simulink model "Demo1"  (R2018b)
settings: Solver=FixedStepDiscrete  StartTime=0.0  StopTime=10  FixedStep=0.0005  RelTol=1e-3  EnableMultiTasking=on
undefined symbols (not defined in the file or in its folder): ADS1, ADS2, br_opening, BRAKE, I_AN06_5V, I_AN08_5V, I_AN09_5V, I_AN10_5V, I_HALL1, I_HALL2, I_SW11_H, I_SW16_H, MnPedal_H, MnPedal_L, MxPedal_H, MxPedal_L, O_PWM1_LS0A7, O_PWM2_LS0A7, O_SW02_LS0A4, O_SW13_HS1A, O_SW14_HS1A, PUMP, th_opening
libraries: ec5744lib x93, canmsglib x14, simulink x5
(part 2 of 2)

== system Demo1/Function-Call Subsystem1/Subsystem ==
  note: 油压范围在500到4500之间
  note: 输出12V高电平给蜂鸣器和待驶指示
      | 灯，启动鸣笛，指示灯亮
  Brake : Inport  OutDataTypeStr=uint16
  Key : Inport  Port=2
  MCU1_rdy : Inport  Port=3
  MCU2_rdy : Inport  Port=4
  1-D Lookup Table2 : Lookup_n-D  NumberOfTableDimensions=1  BreakpointsForDimension1=BRAKE  Table=br_opening  ExtrapMethod=Clip  InternalRulePriority=Speed  OutMin=0  OutMax=100  OutDataTypeStr=uint8  RndMeth=Simplest  InputSameDT=on
  MeaModule3 : ec5744lib/RapidECU_U3/07Calibration/MeaModule  signal=RS
      settings: SourceProductName=ECUCoder for MPC5744
  Terminator : Terminator
  WaitStart&Brake_LED : Stateflow chart  TreatAsAtomicUnit=on
  Break_LED : Outport
  WS_Sig : Outport  Port=2
  WAIT_START : Outport  Port=3
  wires:
  WaitStart&Brake_LED/1(Wait_Start) -> WAIT_START/1  "Wait_Start"
  Brake/1 -> 1-D Lookup Table2/1
  1-D Lookup Table2/1 -> WaitStart&Brake_LED/1(Brake)
  WaitStart&Brake_LED/2(Break_LED) -> Break_LED/1  "Break_LED"
  Key/1 -> WaitStart&Brake_LED/2(Key)
  WaitStart&Brake_LED/3(WS_Sig) -> WS_Sig/1
  WaitStart&Brake_LED/4(RS) -> MeaModule3/1
  MeaModule3/1 -> Terminator/1
  MCU1_rdy/1 -> WaitStart&Brake_LED/3(MCU1_rdy)
  MCU2_rdy/1 -> WaitStart&Brake_LED/4(MCU2_rdy)

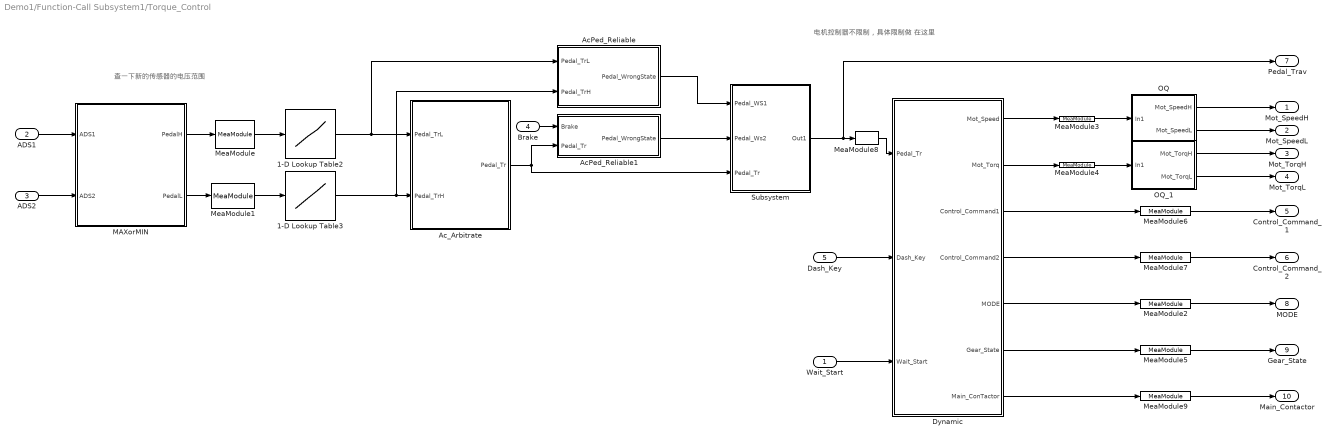
== system Demo1/Function-Call Subsystem1/Torque_Control ==
  note: 查一下新的传感器的电压范围
  note: 电机控制器不限制，具体限制做
      | 在这里
  Wait_Start : Inport
  ADS1 : Inport  Port=2
  ADS2 : Inport  Port=3  OutDataTypeStr=uint16
  "Brake " : Inport  Port=4
  "Dash_Key " : Inport  Port=5  OutMin=0  OutMax=2
  1-D Lookup Table2 : Lookup_n-D  NumberOfTableDimensions=1  BreakpointsForDimension1=ADS1  Table=th_opening  ExtrapMethod=Clip  InternalRulePriority=Speed  OutMin=0  OutMax=95  OutDataTypeStr=uint8  RndMeth=Simplest  InputSameDT=on
  1-D Lookup Table3 : Lookup_n-D  NumberOfTableDimensions=1  BreakpointsForDimension1=ADS2  Table=th_opening  ExtrapMethod=Clip  InternalRulePriority=Speed  OutMin=0  OutMax=95  OutDataTypeStr=uint8  RndMeth=Simplest  InputSameDT=on
  AcPed_Reliable : Stateflow chart  TreatAsAtomicUnit=on
  AcPed_Reliable1 : Stateflow chart  TreatAsAtomicUnit=on
  Ac_Arbitrate : Stateflow chart  TreatAsAtomicUnit=on
  "Dynamic " : Stateflow chart  TreatAsAtomicUnit=on
  MAXorMIN : Subsystem
  MeaModule : ec5744lib/RapidECU_U3/07Calibration/MeaModule  signal=ADSH
      settings: SourceProductName=ECUCoder for MPC5744
  MeaModule1 : ec5744lib/RapidECU_U3/07Calibration/MeaModule  signal=ADSL
      settings: SourceProductName=ECUCoder for MPC5744
  MeaModule2 : ec5744lib/RapidECU_U3/07Calibration/MeaModule  signal=MODE
      settings: SourceProductName=ECUCoder for MPC5744
  MeaModule3 : ec5744lib/RapidECU_U3/07Calibration/MeaModule  signal=MotSpeed
      settings: SourceProductName=ECUCoder for MPC5744
  MeaModule4 : ec5744lib/RapidECU_U3/07Calibration/MeaModule  signal=Mot_torq
      settings: SourceProductName=ECUCoder for MPC5744
  MeaModule5 : ec5744lib/RapidECU_U3/07Calibration/MeaModule  signal=Gear_State
      settings: SourceProductName=ECUCoder for MPC5744
  MeaModule6 : ec5744lib/RapidECU_U3/07Calibration/MeaModule  signal=Control1
      settings: SourceProductName=ECUCoder for MPC5744
  MeaModule7 : ec5744lib/RapidECU_U3/07Calibration/MeaModule  signal=Control2
      settings: SourceProductName=ECUCoder for MPC5744
  MeaModule8 : ec5744lib/RapidECU_U3/07Calibration/MeaModule  signal=c
      settings: SourceProductName=ECUCoder for MPC5744
  MeaModule9 : ec5744lib/RapidECU_U3/07Calibration/MeaModule  signal=Main_Contactor
      settings: SourceProductName=ECUCoder for MPC5744
  OQ : Subsystem
  OQ_1 : Subsystem
  Subsystem : Subsystem
  Mot_SpeedH : Outport
  Mot_SpeedL : Outport  Port=2
  Mot_TorqH : Outport  Port=3
  Mot_TorqL : Outport  Port=4
  "Control_Command_1 " : Outport  Port=5  OutDataTypeStr=uint8
  Control_Command_2 : Outport  Port=6  OutDataTypeStr=uint8
  Pedal_Trav : Outport  Port=7
  MODE : Outport  Port=8
  "Gear_State " : Outport  Port=9
  Main_Contactor : Outport  Port=10
  wires:
  OQ/1(Mot_SpeedH) -> Mot_SpeedH/1
  OQ/2(Mot_SpeedL) -> Mot_SpeedL/1
  OQ_1/1(Mot_TorqH) -> Mot_TorqH/1
  OQ_1/2(Mot_TorqL) -> Mot_TorqL/1
  "Dynamic "/3(Control_Command1) -> MeaModule6/1
  "Dynamic "/4(Control_Command2) -> MeaModule7/1
  "Dash_Key "/1 -> "Dynamic "/2(Dash_Key)
  "Dynamic "/1(Mot_Speed) -> MeaModule3/1
  "Dynamic "/2(Mot_Torq) -> MeaModule4/1
  MeaModule1/1 -> 1-D Lookup Table3/1
  MeaModule/1 -> 1-D Lookup Table2/1
  MeaModule3/1 -> OQ/1(In1)
  MeaModule4/1 -> OQ_1/1(In1)
  MeaModule6/1 -> "Control_Command_1 "/1
  MeaModule7/1 -> Control_Command_2/1
  Ac_Arbitrate/1(Pedal_Tr) -> Subsystem/3(Pedal_Tr), AcPed_Reliable1/2(Pedal_Tr)
  MeaModule8/1 -> "Dynamic "/1(Pedal_Tr)
  Wait_Start/1 -> "Dynamic "/3(Wait_Start)
  "Brake "/1 -> AcPed_Reliable1/1(Brake)
  1-D Lookup Table2/1 -> Ac_Arbitrate/1(Pedal_TrL), AcPed_Reliable/1(Pedal_TrL)
  1-D Lookup Table3/1 -> Ac_Arbitrate/2(Pedal_TrH), AcPed_Reliable/2(Pedal_TrH)
  Subsystem/1(Out1) -> Pedal_Trav/1, MeaModule8/1
  AcPed_Reliable/1(Pedal_WrongState) -> Subsystem/1(Pedal_WS1)
  AcPed_Reliable1/1(Pedal_WrongState) -> Subsystem/2(Pedal_Ws2)
  "Dynamic "/5(MODE) -> MeaModule2/1
  "Dynamic "/6(Gear_State) -> MeaModule5/1
  MeaModule2/1 -> MODE/1
  MeaModule5/1 -> "Gear_State "/1
  "Dynamic "/7(Main_ConTactor) -> MeaModule9/1
  MeaModule9/1 -> Main_Contactor/1
  ADS1/1 -> MAXorMIN/1(ADS1)
  ADS2/1 -> MAXorMIN/2(ADS2)
  MAXorMIN/1("PedalH ") -> MeaModule/1
  MAXorMIN/2(PedalL) -> MeaModule1/1

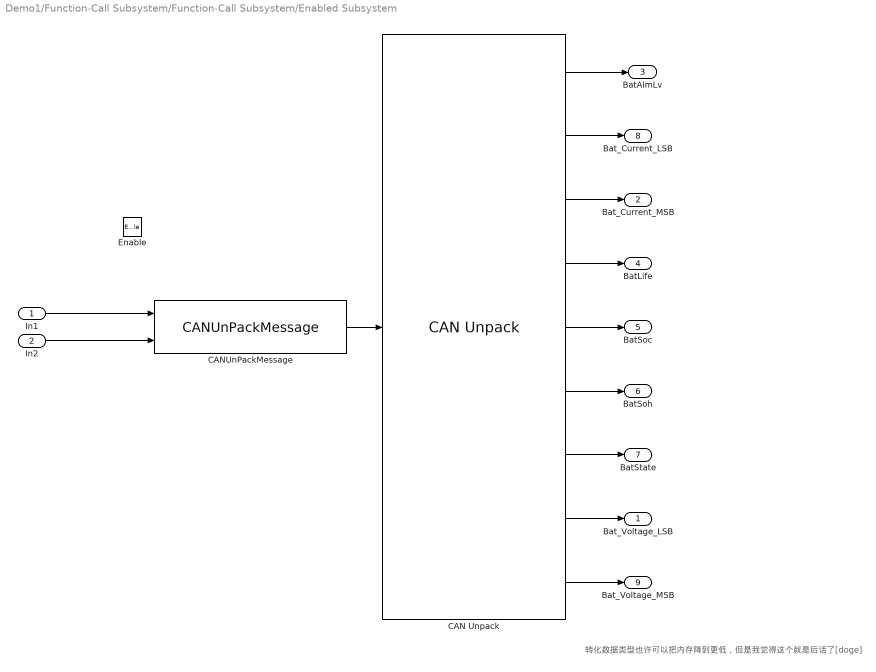
== system Demo1/Function-Call Subsystem/Function-Call Subsystem/Enabled Subsystem ==
  note: 转化数据类型也许可以把内存降到更低，但是我觉得这个就是后话了[doge]
  In1 : Inport
  In2 : Inport  Port=2
  Enable : EnablePort
  CAN Unpack : canmsglib/CAN Unpack  CANdbFile=E:\project\DBC_file\MotControl.dbc  MsgList=BMStoVCU_1  MsgName=BMStoVCU_1  MsgIDType=Extended (29-bit identifier)  MsgIdentifier=408961267  MsgLength=8  SignalInfo=BatAlmLv$52$4$1$2$1$0$1$0$0$15$#BatCurrent_LSB$24$8$1$2$1$0$1$0$0$255$#BatCurrent_MSB$16$8$1$2$1$0$1$0$0$255$#BatLife$56$8$1$2$1$0$1$0$0$255$#BatSoc$32$8$1$2$1$0$1$0$0$255$#BatSoh$40$8$1$2$1$0$1$0$0$255$#BatState$48$4$1$2$1$0$1$0$0$15$#BatVoltage_LSB$8$8$1$2$1$0$1$0$0$255$#BatVoltage_MSB$0$8$1$2$1$0$1$0$0$255$#  NSignals=9  IDPort=off  TimestampPort=off  ErrorPort=off  RemotePort=off  LengthPort=off  StatusPort=off  StartBits=str2num('[int32(52);int32(24);int32(16);int32(56);int32(32);int32(40);int32(48);int32(8);int32(0)]')  SignalSizes=str2num('[int32(4);int32(8);int32(8);int32(8);int32(8);int32(8);int32(4);int32(8);int32(8)]')  ByteOrders=str2num('[int32(1);int32(1);int32(1);int32(1);int32(1);int32(1);int32(1);int32(1);int32(1)]')  DataTypes=str2num('[int32(2);int32(2);int32(2);int32(2);int32(2);int32(2);int32(2);int32(2);int32(2)]')  MultiplexTypes=str2num('[int32(1);int32(1);int32(1);int32(1);int32(1);int32(1);int32(1);int32(1);int32(1)]')  MultiplexValues=str2num('[double(0);double(0);double(0);double(0);double(0);double(0);double(0);double(0);double(0)]')  Factors=str2num('[double(1);double(1);double(1);double(1);double(1);double(1);double(1);double(1);double(1)]')  Offsets=str2num('[double(0);double(0);double(0);double(0);double(0);double(0);double(0);double(0);double(0)]')  Minimums=str2num('[double(0);double(0);double(0);double(0);double(0);double(0);double(0);double(0);double(0)]')  Maximums=str2num('[double(15);double(255);double(255);double(255);double(255);double(255);double(15);double(255);double(255)]')  ApplyMinMax=off
      settings: SourceProductName=Simulink Real-Time  SourceProductBaseCode=XP  DataFormat=CANdb specified signals
  CANUnPackMessage : ec5744lib/RapidECU_U3/04CANCommunication/CANUnPackMessage  datalength=8  canmessagetype=Extended(29-bit ID)  sampletime=-1
      settings: SourceProductName=ECUCoder for MPC5744
  "Bat_Voltage_LSB " : Outport
  Bat_Current_MSB : Outport  Port=2
  "BatAlmLv " : Outport  Port=3
  BatLife : Outport  Port=4
  BatSoc : Outport  Port=5
  BatSoh : Outport  Port=6
  BatState : Outport  Port=7
  Bat_Current_LSB : Outport  Port=8
  "Bat_Voltage_MSB " : Outport  Port=9
  wires:
  CANUnPackMessage/1 -> CAN Unpack/1
  In2/1 -> CANUnPackMessage/2
  In1/1 -> CANUnPackMessage/1
  CAN Unpack/8 -> "Bat_Voltage_LSB "/1
  CAN Unpack/9 -> "Bat_Voltage_MSB "/1
  CAN Unpack/3 -> Bat_Current_MSB/1
  CAN Unpack/1 -> "BatAlmLv "/1
  CAN Unpack/5 -> BatSoc/1
  CAN Unpack/6 -> BatSoh/1
  CAN Unpack/7 -> BatState/1
  CAN Unpack/2 -> Bat_Current_LSB/1
  CAN Unpack/4 -> BatLife/1

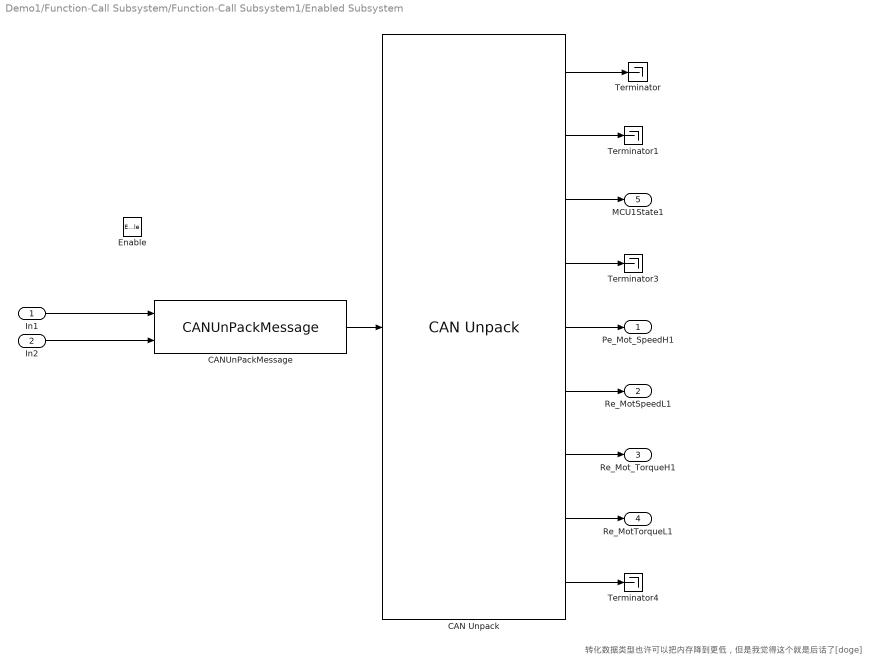
== system Demo1/Function-Call Subsystem/Function-Call Subsystem1/Enabled Subsystem ==
  note: 转化数据类型也许可以把内存降到更低，但是我觉得这个就是后话了[doge]
  In1 : Inport
  In2 : Inport  Port=2
  Enable : EnablePort
  CAN Unpack : canmsglib/CAN Unpack  CANdbFile=E:\project\DBC_file\MotControl.dbc  MsgList=MCU1toVCU_1  MsgName=MCU1toVCU_1  MsgIDType=Extended (29-bit identifier)  MsgIdentifier=218089199  MsgLength=8  SignalInfo=Com_Alarm1$56$2$1$2$1$0$1$0$0$3$#ControlMode_Command1$32$8$1$2$1$0$1$0$0$255$#MCU1State1$40$8$1$2$1$0$1$0$0$255$#MCU1State2$48$2$1$2$1$0$1$0$0$3$#Re_Mot_SpeedH1$8$8$1$2$1$0$1$0$0$255$#Re_Mot_SpeedL1$0$8$1$2$1$0$1$0$0$255$#Re_Mot_TorqueH1$24$8$1$2$1$0$1$0$0$255$#Re_Mot_TorqueL1$16$8$1$2$1$0$1$0$0$255$#Self_Test1$55$1$1$2$1$0$1$0$0$1$#  NSignals=9  IDPort=off  TimestampPort=off  ErrorPort=off  RemotePort=off  LengthPort=off  StatusPort=off  StartBits=str2num('[int32(56);int32(32);int32(40);int32(48);int32(8);int32(0);int32(24);int32(16);int32(55)]')  SignalSizes=str2num('[int32(2);int32(8);int32(8);int32(2);int32(8);int32(8);int32(8);int32(8);int32(1)]')  ByteOrders=str2num('[int32(1);int32(1);int32(1);int32(1);int32(1);int32(1);int32(1);int32(1);int32(1)]')  DataTypes=str2num('[int32(2);int32(2);int32(2);int32(2);int32(2);int32(2);int32(2);int32(2);int32(2)]')  MultiplexTypes=str2num('[int32(1);int32(1);int32(1);int32(1);int32(1);int32(1);int32(1);int32(1);int32(1)]')  MultiplexValues=str2num('[double(0);double(0);double(0);double(0);double(0);double(0);double(0);double(0);double(0)]')  Factors=str2num('[double(1);double(1);double(1);double(1);double(1);double(1);double(1);double(1);double(1)]')  Offsets=str2num('[double(0);double(0);double(0);double(0);double(0);double(0);double(0);double(0);double(0)]')  Minimums=str2num('[double(0);double(0);double(0);double(0);double(0);double(0);double(0);double(0);double(0)]')  Maximums=str2num('[double(3);double(255);double(255);double(3);double(255);double(255);double(255);double(255);double(1)]')  ApplyMinMax=off
      settings: SourceProductName=Simulink Real-Time  SourceProductBaseCode=XP  DataFormat=CANdb specified signals
  CANUnPackMessage : ec5744lib/RapidECU_U3/04CANCommunication/CANUnPackMessage  datalength=8  canmessagetype=Extended(29-bit ID)  sampletime=-1
      settings: SourceProductName=ECUCoder for MPC5744
  Terminator{,1,3..4} (4 alike) : Terminator
  Pe_Mot_SpeedH1 : Outport
  Re_MotSpeedL1 : Outport  Port=2
  Re_Mot_TorqueH1 : Outport  Port=3
  Re_MotTorqueL1 : Outport  Port=4
  MCU1State1 : Outport  Port=5
  wires:
  CAN Unpack/4 -> Terminator3/1
  CAN Unpack/2 -> Terminator1/1
  CAN Unpack/7 -> Re_Mot_TorqueH1/1
  CAN Unpack/6 -> Re_MotSpeedL1/1
  CAN Unpack/5 -> Pe_Mot_SpeedH1/1
  CAN Unpack/1 -> Terminator/1
  CAN Unpack/3 -> MCU1State1/1
  CAN Unpack/9 -> Terminator4/1
  CAN Unpack/8 -> Re_MotTorqueL1/1
  In1/1 -> CANUnPackMessage/1
  In2/1 -> CANUnPackMessage/2
  CANUnPackMessage/1 -> CAN Unpack/1

== system Demo1/Function-Call Subsystem/Function-Call Subsystem1/Subsystem ==
  MCU1_State : Inport
  Chart : Stateflow chart  TreatAsAtomicUnit=on
  Data Type Conversion1 : DataTypeConversion  OutDataTypeStr=uint8
  MeaModule1 : ec5744lib/RapidECU_U3/07Calibration/MeaModule  signal=MCU1_rdy
      settings: SourceProductName=ECUCoder for MPC5744
  MCU1_rdy : Outport
  wires:
  MCU1_State/1 -> Data Type Conversion1/1
  Data Type Conversion1/1 -> Chart/1(MCU1_State)
  Chart/1(MCU1_rdy) -> MeaModule1/1
  MeaModule1/1 -> MCU1_rdy/1

== system Demo1/Function-Call Subsystem/Function-Call Subsystem1/Subsystem1 ==
  DatH : Inport
  DatL : Inport  Port=2
  Chart : Stateflow chart  TreatAsAtomicUnit=on
  Data Type Conversion : DataTypeConversion  OutDataTypeStr=uint16
  Data Type Conversion1 : DataTypeConversion  OutDataTypeStr=uint16
  MeaModule1 : ec5744lib/RapidECU_U3/07Calibration/MeaModule  signal=DC_Bus1
      settings: SourceProductName=ECUCoder for MPC5744
  DC_BusVolt1 : Outport
  wires:
  DatL/1 -> Data Type Conversion/1
  DatH/1 -> Data Type Conversion1/1
  Data Type Conversion/1 -> Chart/2(DC_Bus_VoltL1)
  Data Type Conversion1/1 -> Chart/1(DC_Bus_VoltH1)
  Chart/1(DC_BusVolt1) -> MeaModule1/1
  MeaModule1/1 -> DC_BusVolt1/1

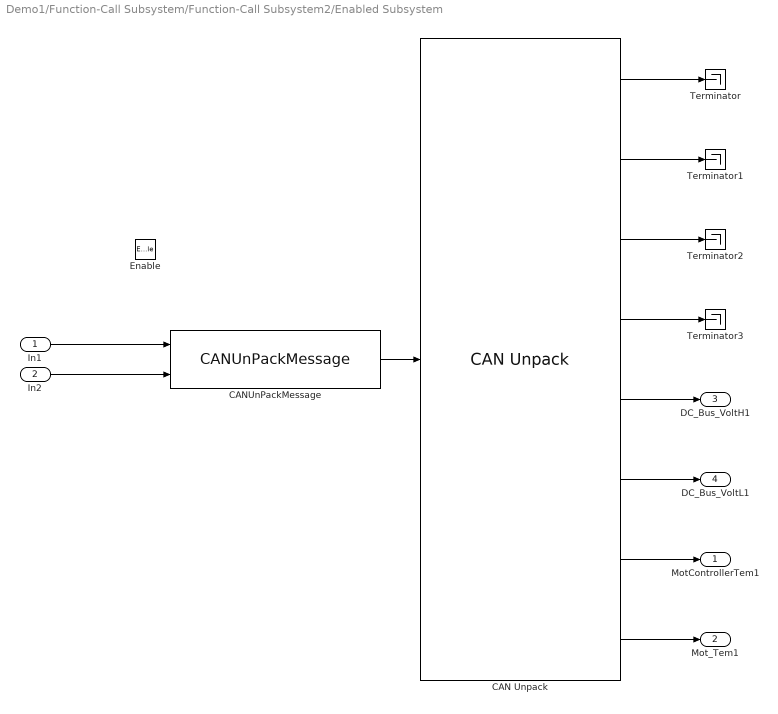
== system Demo1/Function-Call Subsystem/Function-Call Subsystem2/Enabled Subsystem ==
  In1 : Inport
  In2 : Inport  Port=2
  Enable : EnablePort
  CAN Unpack : canmsglib/CAN Unpack  CANdbFile=E:\project\DBC_file\MotControl.dbc  MsgList=MCU1toVCU_2  MsgName=MCU1toVCU_2  MsgIDType=Extended (29-bit identifier)  MsgIdentifier=218089455  MsgLength=8  SignalInfo=AC_CurValidH1$56$8$1$2$1$0$1$0$0$255$#AC_CurValidL1$48$8$1$2$1$0$1$0$0$255$#DC_Bus_CurrH1$40$8$1$2$1$0$1$0$0$255$#DC_Bus_CurrL1$32$8$1$2$1$0$1$0$0$255$#DC_Bus_VoltH1$24$8$1$2$1$0$1$0$0$255$#DC_Bus_VoltL1$16$8$1$2$1$0$1$0$0$255$#MotControllerTem1$0$8$1$2$1$0$1$-50$-50$205$#Mot_Tem1$8$8$1$2$1$0$1$0$0$255$#  NSignals=8  IDPort=off  TimestampPort=off  ErrorPort=off  RemotePort=off  LengthPort=off  StatusPort=off  StartBits=str2num('[int32(56);int32(48);int32(40);int32(32);int32(24);int32(16);int32(0);int32(8)]')  SignalSizes=str2num('[int32(8);int32(8);int32(8);int32(8);int32(8);int32(8);int32(8);int32(8)]')  ByteOrders=str2num('[int32(1);int32(1);int32(1);int32(1);int32(1);int32(1);int32(1);int32(1)]')  DataTypes=str2num('[int32(2);int32(2);int32(2);int32(2);int32(2);int32(2);int32(2);int32(2)]')  MultiplexTypes=str2num('[int32(1);int32(1);int32(1);int32(1);int32(1);int32(1);int32(1);int32(1)]')  MultiplexValues=str2num('[double(0);double(0);double(0);double(0);double(0);double(0);double(0);double(0)]')  Factors=str2num('[double(1);double(1);double(1);double(1);double(1);double(1);double(1);double(1)]')  Offsets=str2num('[double(0);double(0);double(0);double(0);double(0);double(0);double(-50);double(0)]')  Minimums=str2num('[double(0);double(0);double(0);double(0);double(0);double(0);double(-50);double(0)]')  Maximums=str2num('[double(255);double(255);double(255);double(255);double(255);double(255);double(205);double(255)]')  ApplyMinMax=off
      settings: SourceProductName=Simulink Real-Time  SourceProductBaseCode=XP  DataFormat=CANdb specified signals
  CANUnPackMessage : ec5744lib/RapidECU_U3/04CANCommunication/CANUnPackMessage  datalength=8  canmessagetype=Extended(29-bit ID)  sampletime=-1
      settings: SourceProductName=ECUCoder for MPC5744
  Terminator{,1..3} (4 alike) : Terminator
  MotControllerTem1 : Outport
  Mot_Tem1 : Outport  Port=2
  DC_Bus_VoltH1 : Outport  Port=3
  DC_Bus_VoltL1 : Outport  Port=4
  wires:
  CANUnPackMessage/1 -> CAN Unpack/1
  In2/1 -> CANUnPackMessage/2
  In1/1 -> CANUnPackMessage/1
  CAN Unpack/1 -> Terminator/1
  CAN Unpack/3 -> Terminator2/1
  CAN Unpack/2 -> Terminator1/1
  CAN Unpack/5 -> DC_Bus_VoltH1/1
  CAN Unpack/6 -> DC_Bus_VoltL1/1
  CAN Unpack/4 -> Terminator3/1
  CAN Unpack/7 -> MotControllerTem1/1
  CAN Unpack/8 -> Mot_Tem1/1

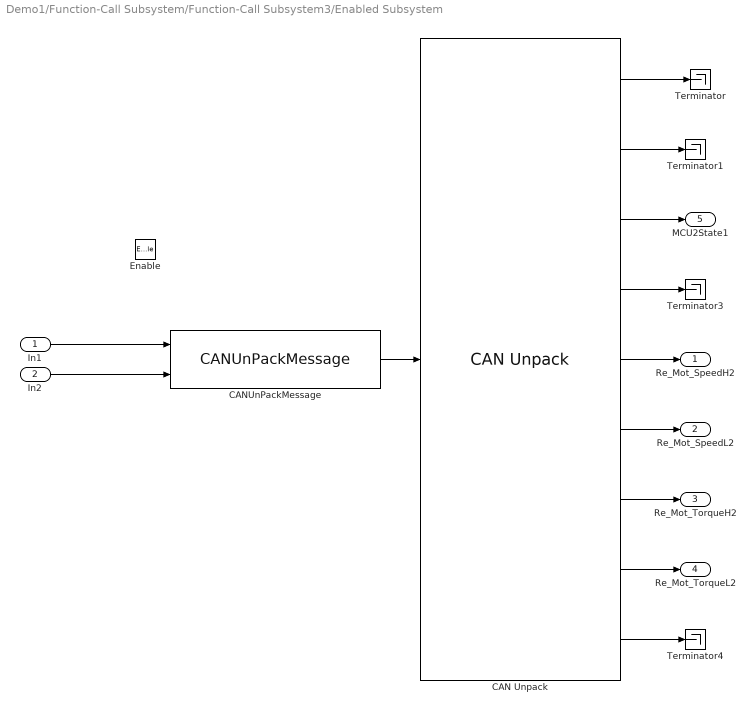
== system Demo1/Function-Call Subsystem/Function-Call Subsystem3/Enabled Subsystem ==
  In1 : Inport
  In2 : Inport  Port=2
  Enable : EnablePort
  CAN Unpack : canmsglib/CAN Unpack  CANdbFile=E:\project\DBC_file\MotControl.dbc  MsgList=MCU2toVCU_1  MsgName=MCU2toVCU_1  MsgIDType=Extended (29-bit identifier)  MsgIdentifier=213000687  MsgLength=8  SignalInfo=Com_Alarm2$56$2$1$2$1$0$1$0$0$3$#ControlMode_Command2$32$8$1$2$1$0$1$0$0$255$#MCU2State1$40$8$1$2$1$0$1$0$0$255$#MCU2State2$48$2$1$2$1$0$1$0$0$3$#Re_Mot_SpeedH2$8$8$1$2$1$0$1$0$-128$127$#Re_Mot_SpeedL2$0$8$1$2$1$0$1$0$-128$127$#Re_Mot_TorqueH2$24$8$1$2$1$0$1$0$0$255$#Re_Mot_TorqueL2$16$8$1$2$1$0$1$0$0$255$#Selt_Test2$55$1$1$2$1$0$1$0$0$1$#  NSignals=9  IDPort=off  TimestampPort=off  ErrorPort=off  RemotePort=off  LengthPort=off  StatusPort=off  StartBits=str2num('[int32(56);int32(32);int32(40);int32(48);int32(8);int32(0);int32(24);int32(16);int32(55)]')  SignalSizes=str2num('[int32(2);int32(8);int32(8);int32(2);int32(8);int32(8);int32(8);int32(8);int32(1)]')  ByteOrders=str2num('[int32(1);int32(1);int32(1);int32(1);int32(1);int32(1);int32(1);int32(1);int32(1)]')  DataTypes=str2num('[int32(2);int32(2);int32(2);int32(2);int32(2);int32(2);int32(2);int32(2);int32(2)]')  MultiplexTypes=str2num('[int32(1);int32(1);int32(1);int32(1);int32(1);int32(1);int32(1);int32(1);int32(1)]')  MultiplexValues=str2num('[double(0);double(0);double(0);double(0);double(0);double(0);double(0);double(0);double(0)]')  Factors=str2num('[double(1);double(1);double(1);double(1);double(1);double(1);double(1);double(1);double(1)]')  Offsets=str2num('[double(0);double(0);double(0);double(0);double(0);double(0);double(0);double(0);double(0)]')  Minimums=str2num('[double(0);double(0);double(0);double(0);double(-128);double(-128);double(0);double(0);double(0)]')  Maximums=str2num('[double(3);double(255);double(255);double(3);double(127);double(127);double(255);double(255);double(1)]')  ApplyMinMax=off
      settings: SourceProductName=Simulink Real-Time  SourceProductBaseCode=XP  DataFormat=CANdb specified signals
  CANUnPackMessage : ec5744lib/RapidECU_U3/04CANCommunication/CANUnPackMessage  datalength=8  canmessagetype=Extended(29-bit ID)  sampletime=-1
      settings: SourceProductName=ECUCoder for MPC5744
  Terminator{,1,3..4} (4 alike) : Terminator
  Re_Mot_SpeedH2 : Outport
  Re_Mot_SpeedL2 : Outport  Port=2
  Re_Mot_TorqueH2 : Outport  Port=3
  Re_Mot_TorqueL2 : Outport  Port=4
  MCU2State1 : Outport  Port=5
  wires:
  In1/1 -> CANUnPackMessage/1
  In2/1 -> CANUnPackMessage/2
  CANUnPackMessage/1 -> CAN Unpack/1
  CAN Unpack/7 -> Re_Mot_TorqueH2/1
  CAN Unpack/4 -> Terminator3/1
  CAN Unpack/6 -> Re_Mot_SpeedL2/1
  CAN Unpack/2 -> Terminator1/1
  CAN Unpack/9 -> Terminator4/1
  CAN Unpack/5 -> Re_Mot_SpeedH2/1
  CAN Unpack/3 -> MCU2State1/1
  CAN Unpack/8 -> Re_Mot_TorqueL2/1
  CAN Unpack/1 -> Terminator/1

== system Demo1/Function-Call Subsystem/Function-Call Subsystem3/Subsystem ==
  MCU2_State : Inport
  Chart : Stateflow chart  TreatAsAtomicUnit=on
  Data Type Conversion1 : DataTypeConversion  OutDataTypeStr=uint8
  MeaModule1 : ec5744lib/RapidECU_U3/07Calibration/MeaModule  signal=MCU2_rdy
      settings: SourceProductName=ECUCoder for MPC5744
  MCU2_rdy : Outport
  wires:
  MCU2_State/1 -> Data Type Conversion1/1
  Data Type Conversion1/1 -> Chart/1(MCU2_State)
  Chart/1(MCU2_rdy) -> MeaModule1/1
  MeaModule1/1 -> MCU2_rdy/1

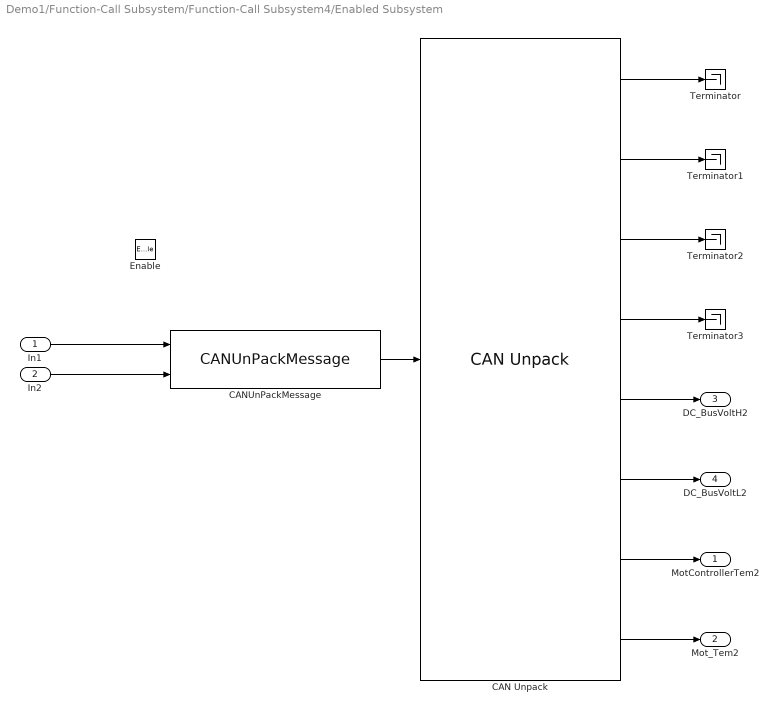
== system Demo1/Function-Call Subsystem/Function-Call Subsystem4/Enabled Subsystem ==
  In1 : Inport
  In2 : Inport  Port=2
  Enable : EnablePort
  CAN Unpack : canmsglib/CAN Unpack  CANdbFile=E:\project\DBC_file\MotControl.dbc  MsgList=MCU2toVCU_2  MsgName=MCU2toVCU_2  MsgIDType=Extended (29-bit identifier)  MsgIdentifier=213066223  MsgLength=8  SignalInfo=AC_CurValidH2$56$8$1$2$1$0$1$0$0$255$#AC_CurValidL2$48$8$1$2$1$0$1$0$0$255$#DC_Bus_CurrH2$40$8$1$2$1$0$1$0$0$255$#DC_Bus_CurrL2$32$8$1$2$1$0$1$0$0$255$#DC_Bus_VoltH2$24$8$1$2$1$0$1$0$0$255$#DC_Bus_VoltL2$16$8$1$2$1$0$1$0$0$255$#MotControllerTem2$0$8$1$2$1$0$1$-50$-50$205$#Mot_Tem2$8$8$1$2$1$0$1$0$0$255$#  NSignals=8  IDPort=off  TimestampPort=off  ErrorPort=off  RemotePort=off  LengthPort=off  StatusPort=off  StartBits=str2num('[int32(56);int32(48);int32(40);int32(32);int32(24);int32(16);int32(0);int32(8)]')  SignalSizes=str2num('[int32(8);int32(8);int32(8);int32(8);int32(8);int32(8);int32(8);int32(8)]')  ByteOrders=str2num('[int32(1);int32(1);int32(1);int32(1);int32(1);int32(1);int32(1);int32(1)]')  DataTypes=str2num('[int32(2);int32(2);int32(2);int32(2);int32(2);int32(2);int32(2);int32(2)]')  MultiplexTypes=str2num('[int32(1);int32(1);int32(1);int32(1);int32(1);int32(1);int32(1);int32(1)]')  MultiplexValues=str2num('[double(0);double(0);double(0);double(0);double(0);double(0);double(0);double(0)]')  Factors=str2num('[double(1);double(1);double(1);double(1);double(1);double(1);double(1);double(1)]')  Offsets=str2num('[double(0);double(0);double(0);double(0);double(0);double(0);double(-50);double(0)]')  Minimums=str2num('[double(0);double(0);double(0);double(0);double(0);double(0);double(-50);double(0)]')  Maximums=str2num('[double(255);double(255);double(255);double(255);double(255);double(255);double(205);double(255)]')  ApplyMinMax=off
      settings: SourceProductName=Simulink Real-Time  SourceProductBaseCode=XP  DataFormat=CANdb specified signals
  CANUnPackMessage : ec5744lib/RapidECU_U3/04CANCommunication/CANUnPackMessage  datalength=8  canmessagetype=Extended(29-bit ID)  sampletime=-1
      settings: SourceProductName=ECUCoder for MPC5744
  Terminator{,1..3} (4 alike) : Terminator
  MotControllerTem2 : Outport
  Mot_Tem2 : Outport  Port=2
  DC_BusVoltH2 : Outport  Port=3
  DC_BusVoltL2 : Outport  Port=4
  wires:
  CANUnPackMessage/1 -> CAN Unpack/1
  In2/1 -> CANUnPackMessage/2
  In1/1 -> CANUnPackMessage/1
  CAN Unpack/3 -> Terminator2/1
  CAN Unpack/1 -> Terminator/1
  CAN Unpack/2 -> Terminator1/1
  CAN Unpack/7 -> MotControllerTem2/1
  CAN Unpack/8 -> Mot_Tem2/1
  CAN Unpack/5 -> DC_BusVoltH2/1
  CAN Unpack/4 -> Terminator3/1
  CAN Unpack/6 -> DC_BusVoltL2/1

== system Demo1/Function-Call Subsystem/Function-Call Subsystem5/Enabled Subsystem ==
  In1 : Inport
  In2 : Inport  Port=2
  Enable : EnablePort
  CAN Unpack : canmsglib/CAN Unpack  CANdbFile=E:\project\DBC_file\MotControl.dbc  MsgList=BMStoVCU_2  MsgName=BMStoVCU_2  MsgIDType=Extended (29-bit identifier)  MsgIdentifier=409092339  MsgLength=8  SignalInfo=CoolingCtl$32$8$1$2$1$0$1$0$0$255$#HeatingCtl$40$8$1$2$1$0$1$0$0$255$#MaxTemp$0$8$1$2$1$0$1$-40$-40$215$#MaxTempNo$16$8$1$2$1$0$1$0$0$255$#MinTemp$8$8$1$2$1$0$1$-40$-40$215$#MinTempNo$24$8$1$2$1$0$1$0$0$255$#  NSignals=6  IDPort=off  TimestampPort=off  ErrorPort=off  RemotePort=off  LengthPort=off  StatusPort=off  StartBits=str2num('[int32(32);int32(40);int32(0);int32(16);int32(8);int32(24)]')  SignalSizes=str2num('[int32(8);int32(8);int32(8);int32(8);int32(8);int32(8)]')  ByteOrders=str2num('[int32(1);int32(1);int32(1);int32(1);int32(1);int32(1)]')  DataTypes=str2num('[int32(2);int32(2);int32(2);int32(2);int32(2);int32(2)]')  MultiplexTypes=str2num('[int32(1);int32(1);int32(1);int32(1);int32(1);int32(1)]')  MultiplexValues=str2num('[double(0);double(0);double(0);double(0);double(0);double(0)]')  Factors=str2num('[double(1);double(1);double(1);double(1);double(1);double(1)]')  Offsets=str2num('[double(0);double(0);double(-40);double(0);double(-40);double(0)]')  Minimums=str2num('[double(0);double(0);double(-40);double(0);double(-40);double(0)]')  Maximums=str2num('[double(255);double(255);double(215);double(255);double(215);double(255)]')  ApplyMinMax=off
      settings: SourceProductName=Simulink Real-Time  SourceProductBaseCode=XP  DataFormat=CANdb specified signals
  CANUnPackMessage : ec5744lib/RapidECU_U3/04CANCommunication/CANUnPackMessage  datalength=8  canmessagetype=Extended(29-bit ID)  sampletime=-1
      settings: SourceProductName=ECUCoder for MPC5744
  "CoolingCtl " : Outport
  HeatingCtl : Outport  Port=2
  MaxTemp : Outport  Port=3
  MaxTempNo : Outport  Port=4
  MinTemp : Outport  Port=5
  MinTempNo : Outport  Port=6
  wires:
  CAN Unpack/4 -> MaxTempNo/1
  CAN Unpack/2 -> HeatingCtl/1
  CAN Unpack/6 -> MinTempNo/1
  CAN Unpack/5 -> MinTemp/1
  CAN Unpack/1 -> "CoolingCtl "/1
  CAN Unpack/3 -> MaxTemp/1
  In1/1 -> CANUnPackMessage/1
  In2/1 -> CANUnPackMessage/2
  CANUnPackMessage/1 -> CAN Unpack/1

== system Demo1/Function-Call Subsystem/Function-Call Subsystem6/Enabled Subsystem ==
  In1 : Inport
  In2 : Inport  Port=2
  Enable : EnablePort
  CAN Unpack : canmsglib/CAN Unpack  CANdbFile=E:\project\DBC_file\MotControl.dbc  MsgList=DashtoVCU  MsgName=DashtoVCU  MsgIDType=Extended (29-bit identifier)  MsgIdentifier=341  MsgLength=8  SignalInfo=Dash_Key$0$8$1$2$1$0$1$0$0$255$#  NSignals=1  IDPort=off  TimestampPort=off  ErrorPort=off  RemotePort=off  LengthPort=off  StatusPort=off  StartBits=str2num('[int32(0)]')  SignalSizes=str2num('[int32(8)]')  ByteOrders=str2num('[int32(1)]')  DataTypes=str2num('[int32(2)]')  MultiplexTypes=str2num('[int32(1)]')  MultiplexValues=str2num('[double(0)]')  Factors=str2num('[double(1)]')  Offsets=str2num('[double(0)]')  Minimums=str2num('[double(0)]')  Maximums=str2num('[double(255)]')  ApplyMinMax=off
      settings: SourceProductName=Simulink Real-Time  SourceProductBaseCode=XP  DataFormat=CANdb specified signals
  CANUnPackMessage : ec5744lib/RapidECU_U3/04CANCommunication/CANUnPackMessage  datalength=8  canmessagetype=Extended(29-bit ID)  sampletime=-1
      settings: SourceProductName=ECUCoder for MPC5744
  Out1 : Outport
  wires:
  CANUnPackMessage/1 -> CAN Unpack/1
  In2/1 -> CANUnPackMessage/2
  In1/1 -> CANUnPackMessage/1
  CAN Unpack/1 -> Out1/1

== system Demo1/Function-Call Subsystem1/Torque_Control/MAXorMIN ==
  ADS1 : Inport
  ADS2 : Inport  Port=2
  Constant1 : Constant  Value=525  OutDataTypeStr=uint16
  Constant2 : Constant  Value=998  OutDataTypeStr=uint16
  Constant6 : Constant  Value=2600  OutDataTypeStr=uint16
  Constant7 : Constant  Value=3200  OutDataTypeStr=uint16
  Switch1 : Switch  Criteria=u2 > Threshold  Threshold=MxPedal_H
  Switch2 : Switch  Criteria=u2 > Threshold  Threshold=MnPedal_H
  Switch3 : Switch  Criteria=u2 > Threshold  Threshold=MxPedal_L
  Switch4 : Switch  Criteria=u2 > Threshold  Threshold=MnPedal_L
  "PedalH " : Outport
  PedalL : Outport  Port=2
  wires:
  Switch3/1 -> Switch4/1, Switch4/2
  Constant1/1 -> Switch4/3
  ADS2/1 -> Switch3/3, Switch3/2
  Switch4/1 -> PedalL/1
  Switch1/1 -> Switch2/1, Switch2/2
  Constant6/1 -> Switch3/1
  Constant2/1 -> Switch2/3
  Constant7/1 -> Switch1/1
  ADS1/1 -> Switch1/3, Switch1/2
  Switch2/1 -> "PedalH "/1

== system Demo1/Function-Call Subsystem1/Torque_Control/OQ ==
  In1 : Inport  OutMin=0  OutMax=10000
  Bitwise Operator : simulink/Logic and Bit Operations/Bitwise Operator  logicop=AND  UseBitMask=on  BitMask=bin2dec('11111111')  BitMaskRealWorld=Stored Integer
  Data Type Conversion : DataTypeConversion  OutDataTypeStr=uint8
  Data Type Conversion1 : DataTypeConversion  OutDataTypeStr=uint8
  Shift Arithmetic : ArithShift  BitShiftNumber=8  BitShiftDirection=Right
  Mot_SpeedH : Outport
  Mot_SpeedL : Outport  Port=2
  wires:
  Shift Arithmetic/1 -> Data Type Conversion/1
  Data Type Conversion/1 -> Mot_SpeedH/1
  Bitwise Operator/1 -> Data Type Conversion1/1
  Data Type Conversion1/1 -> Mot_SpeedL/1
  In1/1 -> Bitwise Operator/1, Shift Arithmetic/1

== system Demo1/Function-Call Subsystem1/Torque_Control/OQ_1 ==
  In1 : Inport
  Bitwise Operator : simulink/Logic and Bit Operations/Bitwise Operator  logicop=AND  UseBitMask=on  BitMask=bin2dec('11111111')  BitMaskRealWorld=Stored Integer
  Data Type Conversion : DataTypeConversion  OutDataTypeStr=uint8
  Data Type Conversion1 : DataTypeConversion  OutDataTypeStr=uint8
  Shift Arithmetic : ArithShift  BitShiftNumber=8  BitShiftDirection=Right
  Mot_TorqH : Outport
  Mot_TorqL : Outport  Port=2
  wires:
  Data Type Conversion1/1 -> Mot_TorqL/1
  Bitwise Operator/1 -> Data Type Conversion1/1
  Data Type Conversion/1 -> Mot_TorqH/1
  Shift Arithmetic/1 -> Data Type Conversion/1
  In1/1 -> Shift Arithmetic/1, Bitwise Operator/1

== system Demo1/Function-Call Subsystem1/Torque_Control/Subsystem ==
  Pedal_WS1 : Inport
  Pedal_Ws2 : Inport  Port=2
  Pedal_Tr : Inport  Port=3
  Constant1 : Constant  Commented=on  Value=0  OutDataTypeStr=uint8
  Constant3 : Constant  Value=0  OutDataTypeStr=uint8
  Logical Operator : Logic  Operator=OR  AllPortsSameDT=off  OutDataTypeStr=boolean
  MeaModule9 : ec5744lib/RapidECU_U3/07Calibration/MeaModule  signal=Pedal_WrongState
      settings: SourceProductName=ECUCoder for MPC5744
  Pedal_Wo_Ar : Switch  Criteria=u2 > Threshold  OutDataTypeStr=uint8
  VCUC_Wo_Ar : Switch  Commented=on  Criteria=u2 > Threshold  OutDataTypeStr=uint8
  Out1 : Outport
  wires:
  MeaModule9/1 -> Pedal_Wo_Ar/2
  Pedal_Ws2/1 -> Logical Operator/2
  Constant3/1 -> Pedal_Wo_Ar/1
  Pedal_Wo_Ar/1 -> Out1/1
  Pedal_WS1/1 -> Logical Operator/1
  Logical Operator/1 -> MeaModule9/1
  Pedal_Tr/1 -> Pedal_Wo_Ar/3
  Constant1/1 -> VCUC_Wo_Ar/1

== stateflow chart Demo1/Function-Call Subsystem1/Torque_Control/AcPed_Reliable ==
  (default) -> (junction 14)
  (junction 14) -> (junction 15) [order 1] : [Pedal_TrL > 100 || Pedal_TrH > 100]
  (junction 14) -> (junction 16) [order 2]
  (junction 15) -> (junction 17) : {Pedal_WrongState = 1;}
  (junction 17) -> (junction 16)
  (junction 16) -> (junction 63)
  (junction 63) -> (junction 64) [order 1] : [Pedal_TrH - Pedal_TrL <= 10 ]
  (junction 63) -> (junction 118) [order 2]
  (junction 64) -> (junction 62) : {Pedal_WrongState = 0;
      | Pedal_WrongCount = 0;}
  (junction 118) -> (junction 85) [order 1] : [Pedal_TrH - Pedal_TrL > 10 ]
  (junction 118) -> (junction 122) [order 2]
  (junction 85) -> (junction 116) : {Pedal_WrongState = 1;}
  (junction 116) -> (junction 65)
  (junction 62) -> (junction 116)
  (junction 65) -> (junction 70)
  (junction 70) -> (junction 71) [order 1] : [Pedal_WrongCount>10]
  (junction 70) -> (junction 72) [order 2]
  (junction 71) -> (junction 73) : {Pedal_WrongState =1;}
  (junction 73) -> (junction 72)
  (junction 72) -> (junction 68)
  data: Pedal_TrL input uint8; Pedal_TrH input uint8; Pedal_WrongState output boolean; Pedal_WrongCount local double

== stateflow chart Demo1/Function-Call Subsystem1/Torque_Control/Dynamic  ==
  state static
    state Norm
      en:
      Control_Command1 = 0;
      Control_Command2 = 0;
      Gear_State = 0;
      MODE = 0;
      Main_ConTactor = 1;
      du:
      Mot_Speed = 2*(0+10000);
      Mot_Torq = 0;
    note: 正常
    state conservation
      en:
      Control_Command1 = 0;
      Control_Command2 = 0;
      Gear_State = 0;
      MODE = 1;
      Main_ConTactor = 1;
      du:
      Mot_Speed = 2*(0+10000);
      Mot_Torq = 0;
    state Sport
      en:
      Mot_Torq = 0;
      Control_Command1 = 0;
      Control_Command2 = 0;
      Gear_State = 0;
      MODE = 2;
      Main_ConTactor = 1;
      du:
      Mot_Speed = 2*(0+10000);
      Mot_Torq = 0;
    note: 节能
    note: 狂暴
    note: 可以在进入精神病模式的时候加入保险机制
    (default) -> static.Norm
    static.Norm -> static.Sport [order 1] : [Dash_Key == 8]
    static.Sport -> static.Norm [order 1] : [Dash_Key == 32]
    static.Norm -> static.conservation [order 2] : [Dash_Key == 16]
    static.conservation -> static.Norm [order 2] : [Dash_Key == 32]
    static.Sport -> static.conservation [order 2] : [Dash_Key == 16]
    static.conservation -> static.Sport [order 1] : [Dash_Key == 8]
  state dynamic
    state Norm
      en:
      Control_Command1 = 2;
      Control_Command2 = 2;
      Gear_State = 2;
      Main_ConTactor = 1;
      du:
      Mot_Speed = 2*(43*Pedal_Tr+10000);
      Mot_Torq = 7.5*Pedal_Tr;
    note: 正常
    state Sport
      en:
      Control_Command1 = 2;
      Control_Command2 = 2;
      Gear_State = 2;
      Main_ConTactor = 1;
      du:
      Mot_Speed = 2*(50*Pedal_Tr+10000);
      Mot_Torq = 8*Pedal_Tr;
    state conservation
      en:
      Control_Command1 = 2;
      Control_Command2 = 2;
      Gear_State = 2;
      Main_ConTactor = 1;
      du:
      Mot_Speed = 2*(30*Pedal_Tr+10000);
      Mot_Torq = 5*Pedal_Tr;
    note: 狂暴
    note: 节能
    (default) -> dynamic.Norm
    dynamic.Norm -> dynamic.Sport [order 1] : [MODE == 2]
    dynamic.Sport -> dynamic.Norm [order 1] : [MODE == 0]
    dynamic.Norm -> dynamic.conservation [order 2] : [MODE == 1]
    dynamic.conservation -> dynamic.Norm [order 1] : [MODE == 0]
    dynamic.Sport -> dynamic.conservation [order 2] : [MODE == 1]
    dynamic.conservation -> dynamic.Sport [order 2] : [MODE == 2]
  (default) -> static
  dynamic -> static : [Wait_Start == 0]
  static -> dynamic : [Wait_Start == 1]
  data: Pedal_Tr input uint8; Dash_Key input double; Mot_Speed output uint16; Mot_Torq output uint16; Control_Command1 output uint8; Control_Command2 output uint8; Wait_Start input boolean; MODE output uint8; Gear_State output double; Main_ConTactor output boolean

== stateflow chart Demo1/Function-Call Subsystem1/Subsystem/WaitStart&Brake_LED ==
  note: /*检测母线电压*/
  note: /*待驾驶*/
  (default) -> (junction 85)
  (junction 85) -> (junction 86) [order 1] : [Brake > 15 ]
  (junction 85) -> (junction 89) [order 2] : {Break_LED = 0;
      | }
  (junction 86) -> (junction 87)
  (junction 87) -> (junction 88) [order 1] : [Key != 0 ]
  (junction 87) -> (junction 90) [order 2] : {Break_LED = 1;}
  (junction 88) -> (junction 91) : {Wait_Start = 1;}
  (junction 90) -> (junction 89)
  (junction 91) -> (junction 90)
  (junction 89) -> (junction 92)
  (junction 92) -> (junction 114) [order 1] : [MCU1_rdy == 0 || MCU2_rdy == 0]
  (junction 92) -> (junction 116) [order 2] : {RS_Rdyfg = 1;
      | }
  (junction 114) -> (junction 115) : {Wait_Start = 0;
      | RS_Rdyfg = 0;
      | }
  (junction 115) -> (junction 116)
  (junction 116) -> (junction 179)
  (junction 179) -> (junction 180) [order 1] : [RS_Rdyfg == 0]
  (junction 180) -> (junction 182) : {RS = 0;}
  (junction 179) -> (junction 181) [order 2]
  (junction 182) -> (junction 181)
  (junction 181) -> (junction 121)
  (junction 121) -> (junction 138) [order 1] : [RS_Rdyfg != 0 && Wait_Start != 0]
  (junction 121) -> (junction 140) [order 2]
  (junction 138) -> (junction 139) : {WS_Sig = 1;
      | RS++;}
  (junction 139) -> (junction 140)
  (junction 140) -> (junction 141)
  (junction 141) -> (junction 147) [order 1] : [RS_Rdyfg != 0 && RS >= 300]
  (junction 141) -> (junction 149) [order 2]
  (junction 147) -> (junction 148) : {WS_Sig = 0;
      | }
  (junction 148) -> (junction 149)
  (junction 149) -> (junction 150)
  data: Brake input uint8; Wait_Start output boolean =0; Key input boolean; Break_LED output boolean; MCU1_rdy input; MCU2_rdy input; WS_Sig output boolean; RS_Rdyfg local double; RS output uint16 =0

== stateflow chart Demo1/Function-Call Subsystem1/Torque_Control/AcPed_Reliable1 ==
  (default) -> (junction 166)
  (junction 166) -> (junction 170) [order 1] : [Pedal_Tr > 10 && Brake > 555]
  (junction 166) -> (junction 167) [order 2] : {Pedal_WrongState = 0;}
  (junction 170) -> (junction 168) : {Pedal_WrongState = 1;}
  (junction 168) -> (junction 167)
  (junction 167) -> (junction 176)
  (junction 176) -> (junction 178) [order 1] : [Pedal_Tr ==0 || Brake ==0]
  (junction 176) -> (junction 180) [order 2] : {Pedal_WrongState = 0;}
  (junction 178) -> (junction 179) : {Pedal_WrongState = 1;}
  (junction 179) -> (junction 180)
  (junction 180) -> (junction 185)
  data: Pedal_WrongState output boolean; Brake input uint16; Pedal_Tr input uint8

== stateflow chart Demo1/Function-Call Subsystem1/Torque_Control/Ac_Arbitrate ==
  (default) -> (junction 14) : /* 油门信号仲裁 */
  (junction 14) -> (junction 15) [order 1] : [Pedal_TrL>Pedal_TrH]
  (junction 14) -> (junction 16) [order 2] : {
      | Pedal_Tr = Pedal_TrL;
      | }
  (junction 15) -> (junction 17) : {
      | Pedal_Tr = Pedal_TrH;
      | }
  (junction 17) -> (junction 16)
  (junction 16) -> (junction 18)
  data: Pedal_TrL input uint8; Pedal_TrH input uint8; Pedal_Tr output uint8

== stateflow chart Demo1/Function-Call Subsystem1/VCU_WrongState ==
  (default) -> (junction 29) : /*当没有报文发送时，标志位有效*/
  (junction 29) -> (junction 31)
  (junction 31) -> (junction 30) [order 1] : [VCULA == 0 || VCULB == 0]
  (junction 31) -> (junction 33) [order 2]
  (junction 30) -> (junction 32) : {CountL++;}
  (junction 32) -> (junction 33)
  (junction 33) -> (junction 39)
  (junction 39) -> (junction 59) [order 1] : [VCULA == 1 || VCULB == 1]
  (junction 39) -> (junction 57) [order 2]
  (junction 59) -> (junction 61) : {CountL = 0;}
  (junction 61) -> (junction 57)
  (junction 57) -> (junction 87)
  (junction 87) -> (junction 88) [order 1] : [VCURA == 0 || VCURB == 0]
  (junction 87) -> (junction 89) [order 2]
  (junction 88) -> (junction 83) : {CountR++;}
  (junction 83) -> (junction 89)
  (junction 89) -> (junction 82)
  (junction 82) -> (junction 90) [order 1] : [VCURA == 1 || VCURB == 1]
  (junction 82) -> (junction 86) [order 2]
  (junction 90) -> (junction 93) : {CountR = 0;}
  (junction 93) -> (junction 86)
  (junction 86) -> (junction 99)
  (junction 99) -> (junction 101) [order 1] : [CountL == 200]
  (junction 99) -> (junction 103) [order 2]
  (junction 101) -> (junction 102) : {CountL = 5;}
  (junction 102) -> (junction 103)
  (junction 103) -> (junction 112)
  (junction 112) -> (junction 116) [order 1] : [CountR == 200]
  (junction 112) -> (junction 110) [order 2]
  (junction 116) -> (junction 115) : {CountR = 5;}
  (junction 115) -> (junction 110)
  (junction 110) -> (junction 66)
  (junction 66) -> (junction 69) [order 1] : [CountL >= 5 && CountR >= 5]
  (junction 66) -> (junction 65) [order 2] : {VCU_Wo = 0;}
  (junction 69) -> (junction 70) : {VCU_Wo = 1;}
  (junction 70) -> (junction 65)
  (junction 65) -> (junction 75)
  data: VCULA input uint8; VCU_Wo output boolean; VCULB input uint8; VCURA input uint8; VCURB input uint8; CountL local uint8 =0; CountR local double =0

== stateflow chart Demo1/Function-Call Subsystem1/BMS_WrongSate ==
  (default) -> (junction 29) : /* 检测到高压上电按钮按下 */
      | /*当没有报文发送时，低边有效*/
  (junction 29) -> (junction 31)
  (junction 31) -> (junction 30) [order 1] : [BMSA == 0 || BMSB == 0]
  (junction 31) -> (junction 33) [order 2]
  (junction 30) -> (junction 32) : {Count ++;}
  (junction 32) -> (junction 33)
  (junction 33) -> (junction 39)
  (junction 39) -> (junction 54) [order 1] : [BMSA == 1 || BMSB == 1]
  (junction 39) -> (junction 56) [order 2]
  (junction 54) -> (junction 55) : {Count = 0;}
  (junction 55) -> (junction 56)
  (junction 56) -> (junction 73)
  (junction 73) -> (junction 75) [order 1] : [Count >= 250]
  (junction 73) -> (junction 77) [order 2]
  (junction 75) -> (junction 76) : {Count =5;}
  (junction 76) -> (junction 77)
  (junction 77) -> (junction 63)
  (junction 63) -> (junction 61) [order 1] : [Count >= 5]
  (junction 63) -> (junction 64) [order 2] : {BMS = 0;}
  (junction 61) -> (junction 66) : {BMS = 1;}
  (junction 66) -> (junction 64)
  (junction 64) -> (junction 71)
  data: BMSA input uint8; BMS output boolean; BMSB input uint8; Count local uint8 =0

== stateflow chart Demo1/Function-Call Subsystem/Function-Call Subsystem1/Subsystem/Chart ==
  state arithmetic
    du:
    MCU1_rdy = 0x01 & MCU1_State;
  (default) -> arithmetic
  data: MCU1_State input; MCU1_rdy output double

== stateflow chart Demo1/Function-Call Subsystem1/Chart1 ==
  state Cal
    du:
    Speed = Gear_NumL/20*2*3.14*0.2286*3.6;
  (default) -> Cal
  data: Gear_NumL input uint16; Gear_NumR input uint16; SpeedL local double; SpeedR local double; Speed output double

== stateflow chart Demo1/Function-Call Subsystem/Function-Call Subsystem3/Subsystem/Chart ==
  state arithmetic
    du:
    MCU2_rdy = 0x01 & MCU2_State;
  (default) -> arithmetic
  data: MCU2_State input; MCU2_rdy output double

== stateflow chart Demo1/Function-Call Subsystem/Function-Call Subsystem1/Subsystem1/Chart ==
  state arithmetic
    du:
    DC_BusVolt1 = (DC_Bus_VoltH1<<8) + DC_Bus_VoltL1;
    DC_BusVolt1 = DC_BusVolt1*0.1;
  (default) -> arithmetic
  data: DC_Bus_VoltH1 input; DC_Bus_VoltL1 input; DC_BusVolt1 output double
